simulink model "swcStopLightsMgr"  (R2022b)
settings: Solver=FixedStepDiscrete  StartTime=0  StopTime=10.0  FixedStep=0.01  RelTol=1e-3
values from neighbouring files (symbols this model uses):
  C1d_stopLightsMgrPriorityTable = Simulink.Parameter    [swcStopLightsMgr_defineIntCalibs.m]
  C_stopLightsEmergencyPeriod = Simulink.Parameter    [swcStopLightsMgr_defineIntCalibs.m]
  C_stopLightsSpeedThresholdSafety = Simulink.Parameter    [swcBrakePedalSignalingApp_defineIntCalibs.m]    (also in swcStopLightsMgr_defineIntCalibs.m)
  CONST_TWO = uint8(2)    [swcStopLightsMgr_defineIntParams.m]
  failureAlert = Simulink.Signal    [swcStopLightsMgr_defineIntCalibs.m]
  Init_FailureAlert = struct('valueState',ValueState.VALUE_STATE_VALID,'failureAlert',FailureAlert.FAILURE_ALERT_NO,'occurrence',uint8(0))    [swcStopLightsMgr_defineIntParams.m]
  Init_lightRequest = struct('Left_lightState',StopLightStateID.STOP_LIGHT_STATE_ID_OFF,'Right_lightState',StopLightStateID.STOP_LIGHT_STATE_ID_OFF,'Middle_lightState',StopLightStateID.STOP_LIGHT_STATE_ID_OFF)    [swcStopLightsMgr_defineIntParams.m]
  Init_setLight = struct('usageId',uint8(0),'LightOut',Init_lightRequest,'requestedPattern',StopLightsPatternID.STOP_LIGHTS_PATTERN_ID_OFF,'isStopLightsOn',false,'BrakeLampStatus',CANBrakeLampStatus.CANBRAKELAMPSTATUS_OFF)    [swcStopLightsMgr_defineIntParams.m]
  Init_StopLightsEvent = struct('valueState',ValueState.VALUE_STATE_VALID,'usageId',uint8(0),'requestedPattern',StopLightsPatternID.STOP_LIGHTS_PATTERN_ID_OFF)    [swcStopLightsMgr_defineIntParams.m]
  Init_switchStopLightState = struct('lightState',StopLightStateID.STOP_LIGHT_STATE_ID_OFF)    [swcStopLightsMgr_defineIntParams.m]
  OCCURRENCE_FALSE = uint8(0)    [swcStopLightsMgr_defineIntParams.m]
  OCCURRENCE_TRUE = uint8(1)    [swcStopLightsMgr_defineIntParams.m]
  PeriodResolution = uint8(20)    [swcStopLightsMgr_defineIntParams.m]
  POWER_AUTHORIZER = uint8(1)    [swcStopLightsMgr_defineIntParams.m]
  STEP_StopLightsMgr = 0.01    [swcStopLightsMgr_defineIntParams.m]
  STOPLIGHTS_IDX = uint8(64)    [swcStopLightsMgr_defineIntParams.m]
  STOPLIGHTS_USAGES_OUTSIDE_WARNING_ON_STRONG_BRAKING = uint8(18)    [swcStopLightsMgr_defineIntParams.m]
  TENMs = uint8(10)    [swcStopLightsMgr_defineIntParams.m]
  USAGEID_DEF = uint8(255)    [swcStopLightsMgr_defineIntParams.m]
  USAGEID_MIN = uint8(0)    [swcStopLightsMgr_defineIntParams.m]
undefined symbols (not defined in the file or in its folder): CANBrakeLampStatus, CANStopLampDiagnosis, occurrence, StopLampDiagnosis, UsageAction, valueState, ValueState
libraries: Ampere_Library x27, simulink x3, KPIT_eBody_Lib_Lighting x1
(part 2 of 2)

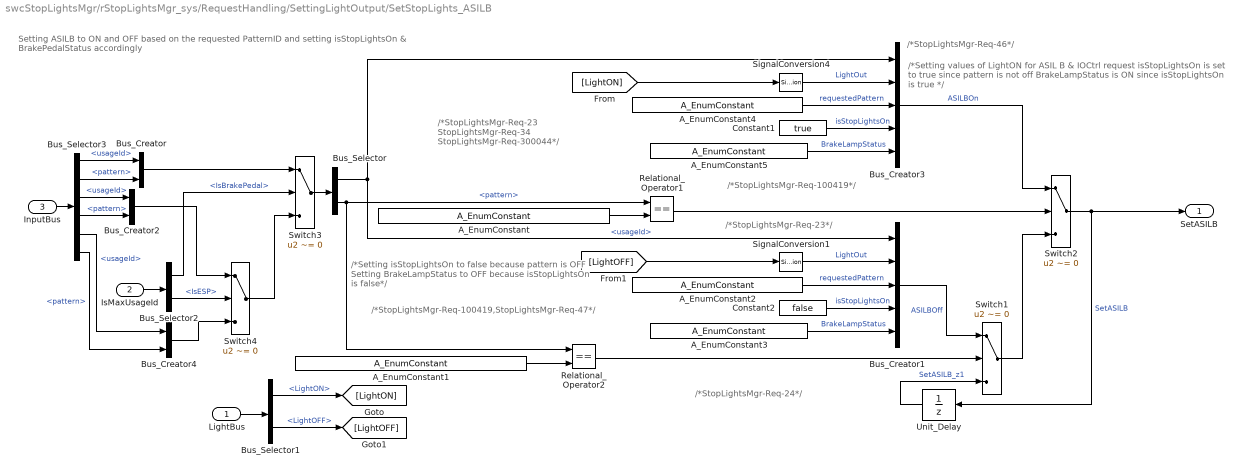
== system swcStopLightsMgr/rStopLightsMgr_sys/RequestHandling/SettingLightOutput/SetStopLights_ASILB ==
  note: /*Setting isStopLightsOn to false because pattern is OFF
      | Setting BrakeLampStatus to OFF because isStopLightsOn is false*/
  note: /*StopLightsMgr-Req-100419,StopLightsMgr-Req-47*/
  note: Setting ASILB to ON and OFF based on the requested PatternID and setting isStopLightsOn & BrakePedalStatus accordingly
  note: /*StopLightsMgr-Req-23
      | StopLightsMgr-Req-34
      | StopLightsMgr-Req-300044*/
  note: /*StopLightsMgr-Req-100419*/
  note: /*StopLightsMgr-Req-23*/
  note: /*StopLightsMgr-Req-24*/
  note: /*StopLightsMgr-Req-46*/
  note: /*Setting values of LightON for ASIL B & IOCtrl request
      | isStopLightsOn is set to true since pattern is not off
      | BrakeLampStatus is ON since isStopLightsOn is true */
  LightBus : Inport
  IsMaxUsageId : Inport  Port=2
  InputBus : Inport  Port=3
  A_EnumConstant : Ampere_Library/User_Defined_Libraries/Sources/A_EnumConstant  Tag=[LIB]  OutDataTypeStr=Enum: StopLightsPatternID  EnumVal=STOP_LIGHTS_PATTERN_ID_ON
      settings: AttributesFormatString=Enum: StopLightsPatternID
  A_EnumConstant1 : Ampere_Library/User_Defined_Libraries/Sources/A_EnumConstant  Tag=[LIB]  OutDataTypeStr=Enum: StopLightsPatternID  EnumVal=STOP_LIGHTS_PATTERN_ID_OFF
      settings: AttributesFormatString=Enum: StopLightsPatternID
  A_EnumConstant2 : Ampere_Library/User_Defined_Libraries/Sources/A_EnumConstant  Tag=[LIB]  OutDataTypeStr=Enum: StopLightsPatternID  EnumVal=STOP_LIGHTS_PATTERN_ID_OFF
      settings: AttributesFormatString=Enum: StopLightsPatternID
  A_EnumConstant3 : Ampere_Library/User_Defined_Libraries/Sources/A_EnumConstant  Tag=[LIB]  OutDataTypeStr=Enum: CANBrakeLampStatus  EnumVal=CANBRAKELAMPSTATUS_OFF
      settings: AttributesFormatString=Enum: CANBrakeLampStatus
  A_EnumConstant4 : Ampere_Library/User_Defined_Libraries/Sources/A_EnumConstant  Tag=[LIB]  OutDataTypeStr=Enum: StopLightsPatternID  EnumVal=STOP_LIGHTS_PATTERN_ID_ON
      settings: AttributesFormatString=Enum: StopLightsPatternID
  A_EnumConstant5 : Ampere_Library/User_Defined_Libraries/Sources/A_EnumConstant  Tag=[LIB]  OutDataTypeStr=Enum: CANBrakeLampStatus  EnumVal=CANBRAKELAMPSTATUS_ON
      settings: AttributesFormatString=Enum: CANBrakeLampStatus
  Bus_Creator : BusCreator  Inputs=2
  Bus_Creator1 : BusCreator  Inputs='usageId','LightOut','requestedPattern','isStopLightsOn','BrakeLampStatus'  OutDataTypeStr=Bus: lightOutput  NonVirtualBus=on
  Bus_Creator2 : BusCreator  Inputs=2
  Bus_Creator3 : BusCreator  Inputs='usageId','LightOut','requestedPattern','isStopLightsOn','BrakeLampStatus'  OutDataTypeStr=Bus: lightOutput  NonVirtualBus=on
  Bus_Creator4 : BusCreator  Inputs=2
  Bus_Selector : BusSelector  OutputSignals=usageId,pattern
  Bus_Selector1 : BusSelector  OutputSignals=LightON,LightOFF
  Bus_Selector2 : BusSelector  OutputSignals=IsBrakePedal,IsESP
  Bus_Selector3 : BusSelector  OutputSignals=BrakePedalStopSignaling_setStopLightsASILB.usageId,BrakePedalStopSignaling_setStopLightsASILB.pattern,ElectronicStabilityControlStopSignaling_setStopLightsASILB.usageId,ElectronicStabilityControlStopSignaling_setStopLightsASILB.pattern,RegenerativeBrakingStopSignaling_setStopLightsASILB.usageId,RegenerativeBrakingStopSignaling_setStopLightsASILB.pattern
  Constant1 : Constant  Value=true
  Constant2 : Constant  Value=false
  Relational_Operator1 : RelationalOperator  Operator===  OutDataTypeStr=boolean  RndMeth=Zero
  Relational_Operator2 : RelationalOperator  Operator===  OutDataTypeStr=boolean  RndMeth=Zero
  SignalConversion1 : SignalConversion  OverrideOpt=off
  SignalConversion4 : SignalConversion  OverrideOpt=off
  Switch{1..4} (4 alike) : Switch  Criteria=u2 ~= 0  RndMeth=Zero  SaturateOnIntegerOverflow=off
  Unit_Delay : UnitDelay  InitialCondition=Init_setLight  SampleTime=-1  HasFrameUpgradeWarning=on
      settings: AttributesFormatString=Init = %<InitialCondition>
  SetASILB : Outport
  wires:
  A_EnumConstant4/1 -> Bus_Creator3/3  "requestedPattern"
  A_EnumConstant5/1 -> Bus_Creator3/5  "BrakeLampStatus"
  Constant1/1 -> Bus_Creator3/4  "isStopLightsOn"
  SignalConversion4/1 -> Bus_Creator3/2  "LightOut"
  [LightON] -> SignalConversion4/1
  A_EnumConstant/1 -> Relational_Operator1/2
  Relational_Operator1/1 -> Switch2/2
  Bus_Creator3/1 -> Switch2/1  "ASILBOn"
  A_EnumConstant1/1 -> Relational_Operator2/2
  Relational_Operator2/1 -> Switch1/2
  Bus_Selector/2 -> Relational_Operator2/1, Relational_Operator1/1  "<pattern>"
  Switch1/1 -> Switch2/3
  Bus_Selector/1 -> Bus_Creator1/1, Bus_Creator3/1  "<usageId>"
  Constant2/1 -> Bus_Creator1/4  "isStopLightsOn"
  SignalConversion1/1 -> Bus_Creator1/2  "LightOut"
  [LightOFF] -> SignalConversion1/1
  A_EnumConstant3/1 -> Bus_Creator1/5  "BrakeLampStatus"
  A_EnumConstant2/1 -> Bus_Creator1/3  "requestedPattern"
  Bus_Creator1/1 -> Switch1/1  "ASILBOff"
  Unit_Delay/1 -> Switch1/3  "SetASILB_z1"
  Switch2/1 -> SetASILB/1, Unit_Delay/1  "SetASILB"
  LightBus/1 -> Bus_Selector1/1
  Bus_Selector1/1 -> [LightON]  "<LightON>"
  Bus_Selector1/2 -> [LightOFF]  "<LightOFF>"
  IsMaxUsageId/1 -> Bus_Selector2/1
  Bus_Selector2/1 -> Switch3/2  "<IsBrakePedal>"
  Bus_Selector3/1 -> Bus_Creator/1  "<usageId>"
  Bus_Selector3/2 -> Bus_Creator/2  "<pattern>"
  InputBus/1 -> Bus_Selector3/1
  Bus_Creator/1 -> Switch3/1
  Bus_Selector2/2 -> Switch4/2  "<IsESP>"
  Bus_Creator2/1 -> Switch4/1
  Switch4/1 -> Switch3/3
  Bus_Selector3/3 -> Bus_Creator2/1  "<usageId>"
  Bus_Selector3/4 -> Bus_Creator2/2  "<pattern>"
  Bus_Creator4/1 -> Switch4/3
  Bus_Selector3/5 -> Bus_Creator4/1  "<usageId>"
  Bus_Selector3/6 -> Bus_Creator4/2  "<pattern>"
  Switch3/1 -> Bus_Selector/1

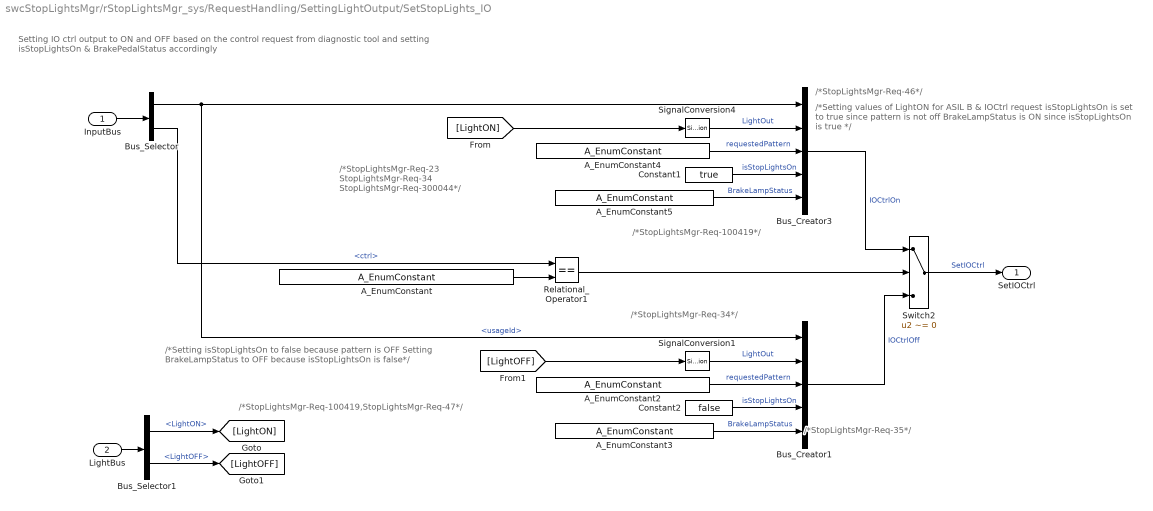
== system swcStopLightsMgr/rStopLightsMgr_sys/RequestHandling/SettingLightOutput/SetStopLights_IO ==
  note: /*Setting isStopLightsOn to false because pattern is OFF
      | Setting BrakeLampStatus to OFF because isStopLightsOn is false*/
  note: /*StopLightsMgr-Req-100419,StopLightsMgr-Req-47*/
  note: Setting IO ctrl output to ON and OFF based on the control request from diagnostic tool and setting isStopLightsOn & BrakePedalStatus accordingly
  note: /*StopLightsMgr-Req-23
      | StopLightsMgr-Req-34
      | StopLightsMgr-Req-300044*/
  note: /*StopLightsMgr-Req-100419*/
  note: /*StopLightsMgr-Req-34*/
  note: /*StopLightsMgr-Req-35*/
  note: /*Setting values of LightON for ASIL B & IOCtrl request
      | isStopLightsOn is set to true since pattern is not off
      | BrakeLampStatus is ON since isStopLightsOn is true */
  note: /*StopLightsMgr-Req-46*/
  InputBus : Inport
  LightBus : Inport  Port=2
  A_EnumConstant : Ampere_Library/User_Defined_Libraries/Sources/A_EnumConstant  Tag=[LIB]  OutDataTypeStr=Enum: IOControlStopLightsRequest  EnumVal=IO_CONTROL_STOPLIGHTS_REQUEST_ON
      settings: AttributesFormatString=Enum: IOControlStopLightsRequest
  A_EnumConstant2 : Ampere_Library/User_Defined_Libraries/Sources/A_EnumConstant  Tag=[LIB]  OutDataTypeStr=Enum: StopLightsPatternID  EnumVal=STOP_LIGHTS_PATTERN_ID_OFF
      settings: AttributesFormatString=Enum: StopLightsPatternID
  A_EnumConstant3 : Ampere_Library/User_Defined_Libraries/Sources/A_EnumConstant  Tag=[LIB]  OutDataTypeStr=Enum: CANBrakeLampStatus  EnumVal=CANBRAKELAMPSTATUS_OFF
      settings: AttributesFormatString=Enum: CANBrakeLampStatus
  A_EnumConstant4 : Ampere_Library/User_Defined_Libraries/Sources/A_EnumConstant  Tag=[LIB]  OutDataTypeStr=Enum: StopLightsPatternID  EnumVal=STOP_LIGHTS_PATTERN_ID_ON
      settings: AttributesFormatString=Enum: StopLightsPatternID
  A_EnumConstant5 : Ampere_Library/User_Defined_Libraries/Sources/A_EnumConstant  Tag=[LIB]  OutDataTypeStr=Enum: CANBrakeLampStatus  EnumVal=CANBRAKELAMPSTATUS_ON
      settings: AttributesFormatString=Enum: CANBrakeLampStatus
  Bus_Creator1 : BusCreator  Inputs='usageId','LightOut','requestedPattern','isStopLightsOn','BrakeLampStatus'  OutDataTypeStr=Bus: lightOutput  NonVirtualBus=on
  Bus_Creator3 : BusCreator  Inputs='usageId','LightOut','requestedPattern','isStopLightsOn','BrakeLampStatus'  OutDataTypeStr=Bus: lightOutput  NonVirtualBus=on
  Bus_Selector : BusSelector  OutputSignals=StopLightsDiag_setStopLightsIOControl.usageId,StopLightsDiag_setStopLightsIOControl.ctrl
  Bus_Selector1 : BusSelector  OutputSignals=LightON,LightOFF
  Constant1 : Constant  Value=true
  Constant2 : Constant  Value=false
  Relational_Operator1 : RelationalOperator  Operator===  OutDataTypeStr=boolean  RndMeth=Zero
  SignalConversion1 : SignalConversion  OverrideOpt=off
  SignalConversion4 : SignalConversion  OverrideOpt=off
  Switch2 : Switch  Criteria=u2 ~= 0  RndMeth=Zero  SaturateOnIntegerOverflow=off
  SetIOCtrl : Outport
  wires:
  A_EnumConstant4/1 -> Bus_Creator3/3  "requestedPattern"
  A_EnumConstant5/1 -> Bus_Creator3/5  "BrakeLampStatus"
  Constant1/1 -> Bus_Creator3/4  "isStopLightsOn"
  InputBus/1 -> Bus_Selector/1
  SignalConversion4/1 -> Bus_Creator3/2  "LightOut"
  [LightON] -> SignalConversion4/1
  A_EnumConstant/1 -> Relational_Operator1/2
  Relational_Operator1/1 -> Switch2/2
  Bus_Creator3/1 -> Switch2/1  "IOCtrlOn"
  Bus_Selector/2 -> Relational_Operator1/1  "<ctrl>"
  Bus_Selector/1 -> Bus_Creator1/1, Bus_Creator3/1  "<usageId>"
  Constant2/1 -> Bus_Creator1/4  "isStopLightsOn"
  SignalConversion1/1 -> Bus_Creator1/2  "LightOut"
  [LightOFF] -> SignalConversion1/1
  A_EnumConstant3/1 -> Bus_Creator1/5  "BrakeLampStatus"
  A_EnumConstant2/1 -> Bus_Creator1/3  "requestedPattern"
  Bus_Creator1/1 -> Switch2/3  "IOCtrlOff"
  Bus_Selector1/2 -> [LightOFF]  "<LightOFF>"
  LightBus/1 -> Bus_Selector1/1
  Bus_Selector1/1 -> [LightON]  "<LightON>"
  Switch2/1 -> SetIOCtrl/1  "SetIOCtrl"

== stateflow chart swcStopLightsMgr/rStopLightsMgr_sys/RequestHandling/SetLightRequest/WarningRequest ==
  note: /*When highest priority request is Warning, Stop lights are turned ON for ONTime and turned OFF for OFFTime indefinitely or turned OFF with UsageId=0*/
  note: /*This flow is added to adhere to AMBDR guidellines IN003*/
  note: /*Setting isStopLightsOn to true becase pattern is not OFF
      | Setting BrakeLampStatus to ON because isStopLightsOn is true*/
  note: /*StopLightsMgr-Req-100419,StopLightsMgr-Req-46*/
  state WarningON
    en:
    LightOut=LightON;
    usageId=STOPLIGHTS_USAGES_OUTSIDE_WARNING_ON_STRONG_BRAKING;
    requestedPattern=STOP_LIGHTS_PATTERN_ID_WARNING;
    isStopLightsOn=true;
    BrakeLampStatus=CANBRAKELAMPSTATUS_ON;
    ONTime = (C_stopLightsEmergencyPeriod * PeriodResolution)/(CONST_TWO* TENMs);
    note: /*StopLightsMgr-Req-300043,StopLightsMgr-Req-45*/
  state WarningOFF
    en:
    LightOut=LightOFF;
    usageId=STOPLIGHTS_USAGES_OUTSIDE_WARNING_ON_STRONG_BRAKING;
    requestedPattern=STOP_LIGHTS_PATTERN_ID_WARNING;
    isStopLightsOn=true;
    BrakeLampStatus=CANBRAKELAMPSTATUS_ON;
    OFFTime = (C_stopLightsEmergencyPeriod * PeriodResolution)/(CONST_TWO* TENMs);
    note: /*StopLightsMgr-Req-300043,StopLightsMgr-Req-45*/
  state NoAuthorization
    en:
    LightOut=LightOFF;
    usageId=POWER_AUTHORIZER;
    requestedPattern=STOP_LIGHTS_PATTERN_ID_OFF;
    isStopLightsOn=false;
    BrakeLampStatus=CANBRAKELAMPSTATUS_OFF;
  note: /* Output arbitrated when authorization is not present*/
  note: /*StopLightsMgr-Req-37,StopLightsMgr-Req-39*/
  (default) -> (junction 80)
  (junction 80) -> (junction 77) [order 1] : % Initializing buses due to SF bug
      | [InitBusInFlowChart==false]
  (junction 80) -> (junction 81) [order 2]
  (junction 77) -> (junction 76) : {InitBusInFlowChart=true;
      | LightOut=Init_lightRequest;}
  (junction 76) -> (junction 81)
  (junction 81) -> (junction 7)
  WarningOFF -> WarningON [order 2] : [after(OFFTime, tick)]
  (junction 7) -> WarningON [order 1] : [Warning_Authorized && IsWarning]
  NoAuthorization -> (junction 7)
  (junction 7) -> NoAuthorization [order 2]
  WarningON -> WarningOFF [order 2] : [after(ONTime, tick)]
  WarningON -> NoAuthorization [order 1] : [!(Warning_Authorized) || !(IsWarning)]
  WarningOFF -> NoAuthorization [order 1] : [!(Warning_Authorized) || !(IsWarning)]
  data: Warning_Authorized input; usageId output uint8 =USAGEID_MIN; LightOut output Bus: lightRequest; IsWarning input; LightON input Bus: lightRequest; LightOFF input Bus: lightRequest; requestedPattern output Enum: StopLightsPatternID =StopLightsPatternID.STOP_LIGHTS_PATTERN_ID_OFF; isStopLightsOn output boolean =false; C_stopLightsEmergencyPeriod parameter; STOPLIGHTS_USAGES_OUTSIDE_WARNING_ON_STRONG_BRAKING parameter; ONTime local uint8 =INIT_TIME; OFFTime local uint8 =INIT_TIME; TENMs parameter; CONST_TWO parameter; PeriodResolution parameter; BrakeLampStatus output Enum: CANBrakeLampStatus =CANBrakeLampStatus.CANBRAKELAMPSTATUS_OFF; POWER_AUTHORIZER parameter; Init_lightRequest parameter Bus: lightRequest; InitBusInFlowChart local boolean =false
